simulink model "gyroModulationsExampleSim"  (R2019b)
settings: Solver=FixedStepAuto  StartTime=0.0  StopTime=final_time  FixedStep=step_time  RelTol=1e-3
values from neighbouring files (symbols this model uses):
  ang_vel = ang_vel*pi/180    (= 0.174532925199)    [gyroControlDemod.m]    (also in gyroControlPhaseUnmod.m; gyroDigControlDemod.m; gyroModulationsExample.m = 0.314159265359; gyroSakajiri2008.m)
  f_mod = 1/(2*tau)    (= 109039.379296)    [gyroControlDemod.m]    (also in gyroControlPhaseUnmod.m; gyroDigControlDemod.m; gyroModulationsExample.m; gyroSakajiri2008.m)
  I0 = 1    [gyroControlDemod.m]    (also in gyroControlPhaseUnmod.m; gyroDigControlDemod.m; gyroModulationsExample.m; gyroSakajiri2008.m)
  mod_amp = (op/2)/mod_sf    (= 0.875)    [gyroControlDemod.m]    (also in gyroControlPhaseUnmod.m; gyroDigControlDemod.m; gyroModulationsExample.m; gyroSakajiri2008.m)
  mod_sf = pi/mod_vpi    (= 0.897597901026)    [gyroControlDemod.m]    (also in gyroControlPhaseUnmod.m; gyroDigControlDemod.m; gyroModulationsExample.m; gyroSakajiri2008.m)
  mod_signal = 4    [gyroModulationsExample.m]
  pd_resp = 1    [gyroControlDemod.m]    (also in gyroControlPhaseUnmod.m; gyroDigControlDemod.m; gyroModulationsExample.m; gyroSakajiri2008.m)
  sf = 2*pi*L*D/(lambda*c)    [gyroControlDemod.m]    (also in gyroControlPhaseUnmod.m; gyroDigControlDemod.m; gyroModulationsExample.m; gyroSakajiri2008.m)
  step_time = tau/10    (= 4.58549932353e-07)    [gyroControlDemod.m]    (also in gyroControlPhaseUnmod.m = 2.29274966176e-06; gyroDigControlDemod.m = 2.29274966176e-06; gyroModulationsExample.m = 4.58549932353e-08; gyroSakajiri2008.m = 1.14637483088e-07)
  tau = L/v    (= 4.58549932353e-06)    [gyroControlDemod.m]    (also in gyroControlPhaseUnmod.m; gyroDigControlDemod.m; gyroModulationsExample.m; gyroSakajiri2008.m)
libraries: simulink x1, powerlib_meascontrol x1
settings Model: Creator=Stinky  LastModifiedBy=Stinky

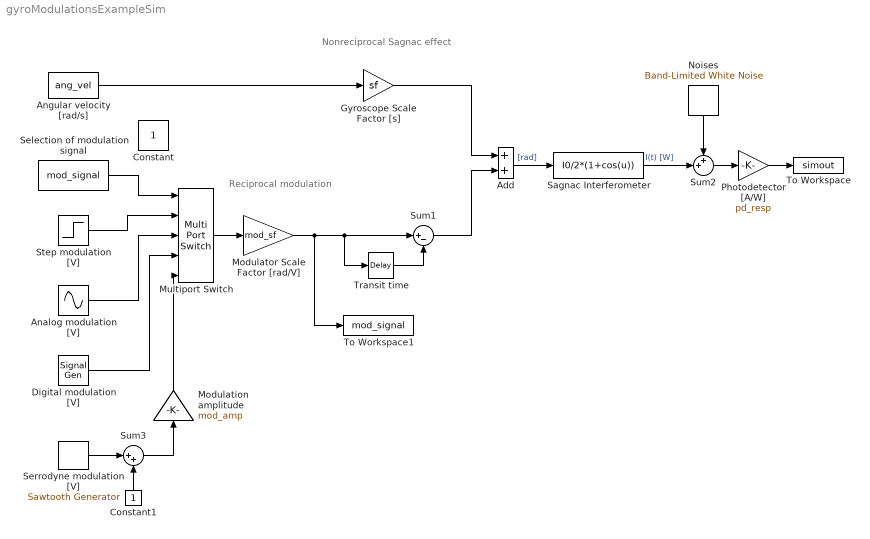
== system gyroModulationsExampleSim ==
  note: Nonreciprocal
      | Sagnac effect
  note: Reciprocal modulation
  Add : Sum
  Analog modulation [V] : Sin  Amplitude=mod_amp  Frequency=2*pi*f_mod  SampleTime=0
  Angular velocity [rad/s] : Constant  Value=ang_vel
  Constant1 : Constant
  Digital modulation [V] : SignalGenerator  WaveForm=square  Amplitude=mod_amp  Frequency=f_mod/2
  Gyroscope Scale Factor [s] : Gain  Gain=sf
  Modulation amplitude : Gain  Gain=mod_amp
  Modulator Scale Factor [rad/V] : Gain  Gain=mod_sf
  Multiport Switch : MultiPortSwitch  Inputs=4
  Noises : simulink/Sources/Band-Limited White Noise  Cov=1e-14  Ts=step_time  seed=[23341]
  Photodetector [A/W] : Gain  Gain=pd_resp
  Sagnac Interferometer : Fcn  Expr=I0/2*(1+cos(u))
  Selection of modulation signal : Constant  Value=mod_signal
  Serrodyne modulation [V] : powerlib_meascontrol/Pulse & Signal Generators/Sawtooth Generator  Freq=f_mod  Phase=180  Ts=0
      settings: SourceProductName=Simscape Electrical
  Step modulation [V] : Step  Time=tau  After=mod_amp  SampleTime=0
  Sum1 : Sum  Inputs=|+-
  Sum2 : Sum  Inputs=++|
  Sum3 : Sum  Inputs=|++
  To Workspace : ToWorkspace  VariableName=simout  SaveFormat=Timeseries  SampleTime=-1
  To Workspace1 : ToWorkspace  VariableName=mod_signal  SaveFormat=Timeseries  SampleTime=-1
  Transit time : TransportDelay  DelayTime=tau
  Constant : Constant  IOType=siggen
  wires:
  Gyroscope Scale Factor [s]/1 -> Add/1
  Add/1 -> Sagnac Interferometer/1  "[rad]"
  Transit time/1 -> Sum1/2
  Sum1/1 -> Add/2
  Angular velocity [rad/s]/1 -> Gyroscope Scale Factor [s]/1
  Modulator Scale Factor [rad/V]/1 -> To Workspace1/1, Sum1/1, Transit time/1
  Photodetector [A/W]/1 -> To Workspace/1
  Sum2/1 -> Photodetector [A/W]/1
  Step modulation [V]/1 -> Multiport Switch/2
  Analog modulation [V]/1 -> Multiport Switch/3
  Selection of modulation signal/1 -> Multiport Switch/1
  Digital modulation [V]/1 -> Multiport Switch/4
  Serrodyne modulation [V]/1 -> Sum3/1
  Sum3/1 -> Modulation amplitude/1
  Constant1/1 -> Sum3/2
  Multiport Switch/1 -> Modulator Scale Factor [rad/V]/1
  Modulation amplitude/1 -> Multiport Switch/5
  Sagnac Interferometer/1 -> Sum2/2  "I(t) [W]"
  Noises/1 -> Sum2/1
